simulink model "PIDControllerSuspensionSimulink"  (R2020a)
settings: Solver=VariableStepAuto  StartTime=0.0  StopTime=10.0  RelTol=1e-3
values from neighbouring files (symbols this model uses):
  b = 10    [MassSpringDamper_PID_Run.m]
  F = 1    [MassSpringDamper_PID_Run.m]
  k = 20    [MassSpringDamper_PID_Run.m]
  Kd = 200    [MassSpringDamper_PID_Run.m]
  Ki = 400    [MassSpringDamper_PID_Run.m]
  Kp = 500    [MassSpringDamper_PID_Run.m]
  M = 1    [MassSpringDamper_PID_Run.m]
settings Model: Creator=diogo  LastModifiedBy=diogo

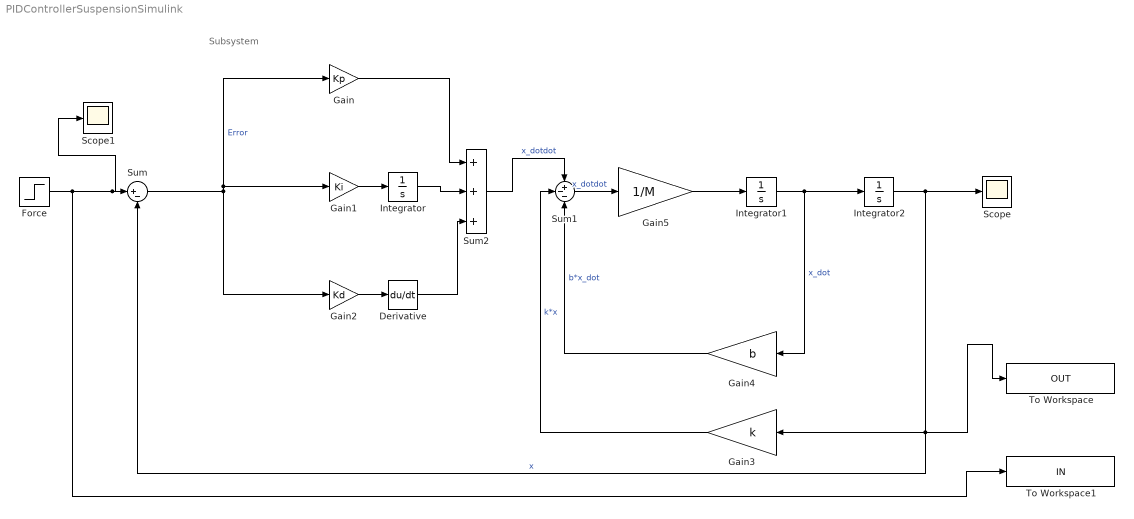
== system PIDControllerSuspensionSimulink ==
  note: Subsystem
  Derivative : Derivative
  Force : Step  After=F  SampleTime=0
  Gain : Gain  Gain=Kp
  Gain1 : Gain  Gain=Ki
  Gain2 : Gain  Gain=Kd
  Gain3 : Gain  Gain=k
  Gain4 : Gain  Gain=b
  Gain5 : Gain  Gain=1/M
  Integrator : Integrator
  Integrator1 : Integrator
  Integrator2 : Integrator
  Scope : Scope
  Scope1 : Scope
  Sum : Sum  Inputs=|+-
  Sum1 : Sum  Inputs=+--
  Sum2 : Sum  Inputs=+++
  To Workspace : ToWorkspace  VariableName=OUT  SampleTime=-1
      settings: Save2DSignal=2-D array (concatenate along first dimension)
  To Workspace1 : ToWorkspace  VariableName=IN  SampleTime=-1
      settings: Save2DSignal=2-D array (concatenate along first dimension)
  wires:
  Gain4/1 -> Sum1/3  "b*x_dot"
  Integrator1/1 -> Gain4/1, Integrator2/1  "x_dot"
  Gain5/1 -> Integrator1/1
  Integrator2/1 -> Scope/1, To Workspace/1, Sum/2, Gain3/1  "x"
  Force/1 -> To Workspace1/1, Scope1/1, Sum/1
  Sum1/1 -> Gain5/1  "x_dotdot"
  Gain3/1 -> Sum1/2  "k*x"
  Sum/1 -> Gain1/1, Gain/1, Gain2/1  "Error"
  Derivative/1 -> Sum2/3
  Gain1/1 -> Integrator/1
  Gain/1 -> Sum2/1
  Integrator/1 -> Sum2/2
  Gain2/1 -> Derivative/1
  Sum2/1 -> Sum1/1  "x_dotdot"
